simulink model "random_carrier_triangular"  (R2013b)
settings: Solver=ode45  StartTime=0.0  StopTime=1  RelTol=1e-3
libraries: powerlib_meascontrol x1
settings Model: Creator=User  LastModifiedBy=User

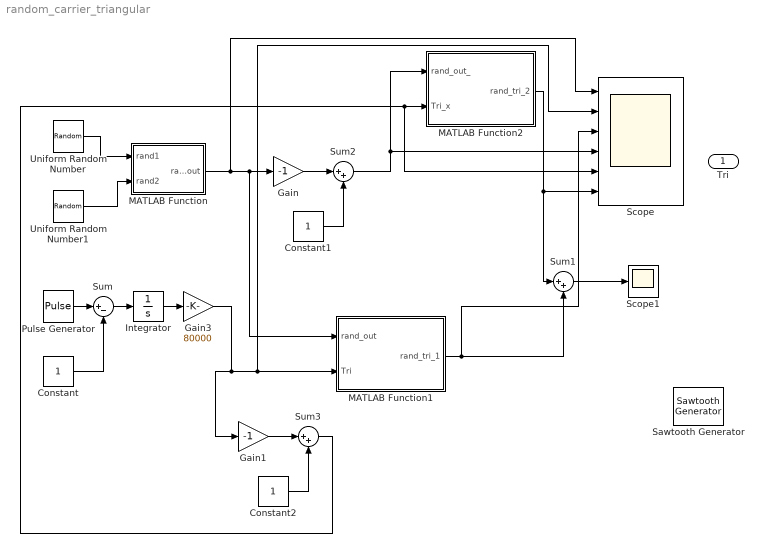
== system random_carrier_triangular ==
  Constant : Constant
  Constant1 : Constant
  Constant2 : Constant
  Gain : Gain  Gain=-1
  Gain1 : Gain  Gain=-1
  Gain3 : Gain  Gain=80000
  Integrator : Integrator
  MATLAB Function : MATLAB Function  TreatAsAtomicUnit=on
  MATLAB Function1 : MATLAB Function  TreatAsAtomicUnit=on
  MATLAB Function2 : MATLAB Function  TreatAsAtomicUnit=on
  Pulse Generator : DiscretePulseGenerator  PulseType=Time based  Amplitude=2  Period=1/40000  PulseWidth=50
  Sawtooth Generator : powerlib_meascontrol/Pulse & Signal Generators/Sawtooth Generator  Freq=1e3  Phase=180  Ts=0
  Scope : Scope  NumInputPorts=6
      settings: YMin=-0.1~-5~-0.1~-0.1~-0.1~-5  YMax=1.1~5~1.1~1.1~1.1~5
  Scope1 : Scope
  Sum : Sum  Inputs=|+-
  Sum1 : Sum  Inputs=|++
  Sum2 : Sum  Inputs=|++
  Sum3 : Sum  Inputs=|++
  Uniform Random Number : UniformRandomNumber  Minimum=0  Seed=1  SampleTime=0.000025
  Uniform Random Number1 : UniformRandomNumber  Minimum=0  SampleTime=0.000025
  Tri : Outport
  wires:
  Uniform Random Number/1 -> MATLAB Function/1(rand1)
  Uniform Random Number1/1 -> MATLAB Function/2(rand2)
  Sum/1 -> Integrator/1
  Pulse Generator/1 -> Sum/1
  Constant/1 -> Sum/2
  Integrator/1 -> Gain3/1
  MATLAB Function/1(rand_out) -> Scope/1, MATLAB Function1/1(rand_out), Gain/1
  Gain/1 -> Sum2/1
  Constant1/1 -> Sum2/2
  Gain3/1 -> MATLAB Function1/2(Tri), Scope/2, Gain1/1
  Sum2/1 -> Scope/4, MATLAB Function2/1(rand_out_)
  Gain1/1 -> Sum3/1
  Constant2/1 -> Sum3/2
  MATLAB Function2/1(rand_tri_2) -> Scope/6, Sum1/1
  MATLAB Function1/1(rand_tri_1) -> Scope/3, Sum1/2
  Sum1/1 -> Scope1/1
  Sum3/1 -> Scope/5, MATLAB Function2/2(Tri_x)

== matlab function random_carrier_triangular/MATLAB Function1 ==
  data: rand_out input; Tri input; rand_tri_1 output
function rand_tri_1  = fcn(rand_out,Tri)
rand_tri_1 = 0;
if (rand_out==1)
    rand_tri_1=Tri;
end

== matlab function random_carrier_triangular/MATLAB Function ==
  data: rand1 input; rand_out output; rand2 input
function rand_out = fcn(rand1,rand2)
rand_out = 0;
if (rand1>=rand2)
    rand_out=1;
else
    rand_out=0;
end;

== matlab function random_carrier_triangular/MATLAB Function2 ==
  data: rand_out_ input; Tri_x input; rand_tri_2 output
function rand_tri_2  = fcn(rand_out_,Tri_x)
rand_tri_2 = 0;
if (rand_out_==1)
    rand_tri_2=Tri_x;
else
    rand_tri_2=0;
end
